simulink model "DDPG"  (R2023a)
settings: Solver=VariableStepAuto  StartTime=0.0  StopTime=10  FixedStep=0.002  RelTol=1e-3
values from neighbouring files (symbols this model uses):
  A = [0 1 0 -1 ... (first row only)    [DDPG_TRAIN.m]
  B = [0; 1/ms; 0; -1/mus]    [DDPG_TRAIN.m]
  B1 = [0; 0; -1; cus/mus]    [DDPG_TRAIN.m]
  C = [1 0 0 0 ... (first row only)    [DDPG_TRAIN.m]
  D = [0; 1/ms]    [DDPG_TRAIN.m]
  Ts = 0.2    [DDPG_TRAIN.m]
undefined symbols (not defined in the file or in its folder): DiscIntNeverNeededParam
libraries: simulink x4, rllib x1
settings Model: Creator=msalm  LastModifiedBy=msalm
settings DataIOCC: ReturnWorkspaceOutputs=off
settings DebuggingCC: AlgebraicLoopMsg=none

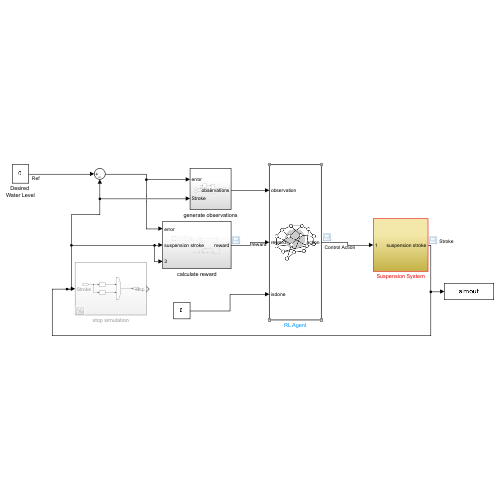
[thumbnail: Simulink's stored preview of the top-level diagram]
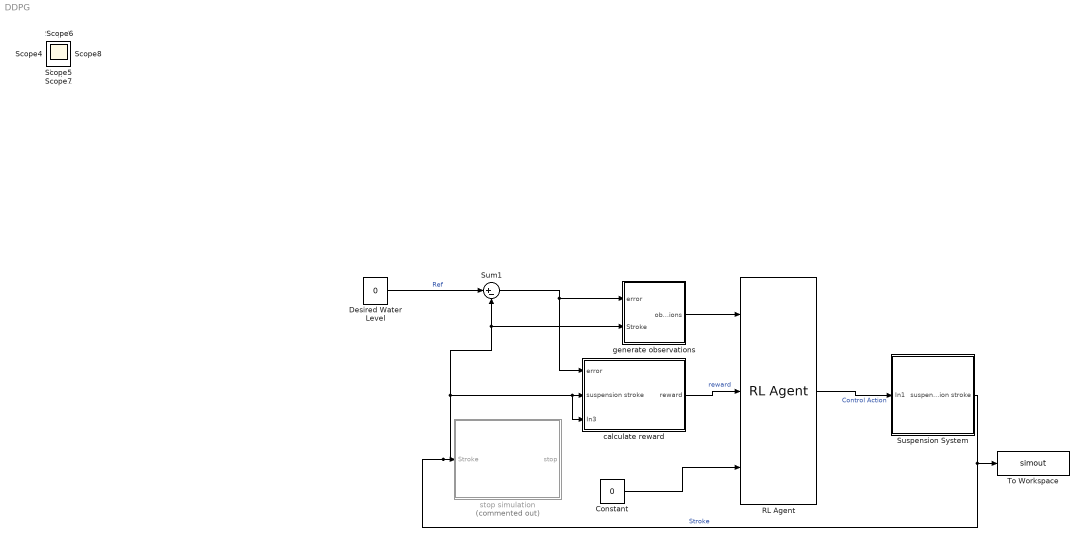
== system DDPG ==
  Constant : Constant  Value=0
  Desired Water Level : Constant  Value=0
  RL Agent : rllib/RL Agent  Agent=agent  ExternalActionAsInput=off  ProvideLastAction=off  ProvideCumRwd=off  TreatAsDirectFeedthrough=on  UseStrictObservationDataTypes=off
  Sum1 : Sum  Inputs=|+-  SaturateOnIntegerOverflow=on
  Suspension System : Subsystem
  To Workspace : ToWorkspace  VariableName=simout  SaveFormat=Timeseries  SampleTime=-1
  calculate reward : Subsystem
  generate observations : Subsystem
  stop simulation : Subsystem  Commented=on
  Scope{,1..8} (9 alike) : Scope
  wires:
  generate observations/1(observations) -> RL Agent/1
  calculate reward/1(reward) -> RL Agent/2  "reward"
  RL Agent/1 -> Suspension System/1(In1)  "Control Action"
  Sum1/1 -> calculate reward/1(error), generate observations/1(error)
  Suspension System/1(suspension stroke) -> stop simulation/1(Stroke), Sum1/2, generate observations/2(Stroke), calculate reward/3(In3), calculate reward/2(suspension stroke), To Workspace/1  "Stroke"
  Desired Water Level/1 -> Sum1/1  "Ref"
  Constant/1 -> RL Agent/3

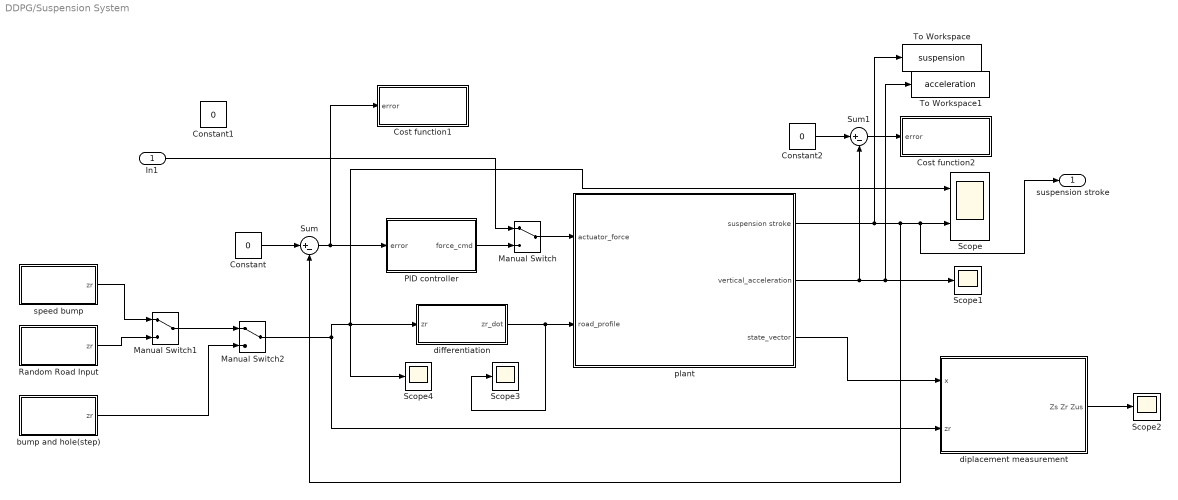
== system DDPG/Suspension System ==
  In1 : Inport
  Constant : Constant  Value=0
  Constant1 : Constant  Value=0
  Constant2 : Constant  Value=0
  Cost function1 : Subsystem
  Cost function2 : Subsystem
  Manual Switch : ManualSwitch
  Manual Switch1 : ManualSwitch
  Manual Switch2 : ManualSwitch
  PID controller : Subsystem
  Random Road Input : Subsystem
  Scope : Scope  NumInputPorts=2
  Scope{1..4} (4 alike) : Scope
  Sum : Sum  Inputs=|+-
  Sum1 : Sum  Inputs=|+-
  To Workspace : ToWorkspace  VariableName=suspension  SampleTime=-1
  To Workspace1 : ToWorkspace  VariableName=acceleration  SampleTime=-1
  bump and hole(step) : Subsystem
  differentiation : Subsystem
  diplacement measurement : Subsystem
  plant : Subsystem
  speed bump : Subsystem
  suspension stroke : Outport
  wires:
  Manual Switch1/1 -> Manual Switch2/1
  plant/3(state_vector) -> diplacement measurement/1(x)
  Random Road Input/1(zr) -> Manual Switch1/2
  Sum1/1 -> Cost function2/1(error)
  Constant2/1 -> Sum1/1
  diplacement measurement/1(Zs Zr Zus) -> Scope2/1
  Constant/1 -> Sum/1
  Sum/1 -> Cost function1/1(error), PID controller/1(error)
  PID controller/1(force_cmd) -> Manual Switch/2
  plant/1(suspension stroke) -> To Workspace/1, Sum/2, suspension stroke/1, Scope/2
  plant/2(vertical_acceleration) -> To Workspace1/1, Scope1/1, Sum1/2
  differentiation/1(zr_dot) -> Scope3/1, plant/2(road_profile)
  Manual Switch/1 -> plant/1(actuator_force)
  bump and hole(step)/1(zr) -> Manual Switch2/2
  speed bump/1(zr) -> Manual Switch1/1
  In1/1 -> Manual Switch/1
  Manual Switch2/1 -> diplacement measurement/2(zr), Scope4/1, Scope/1, differentiation/1(zr)

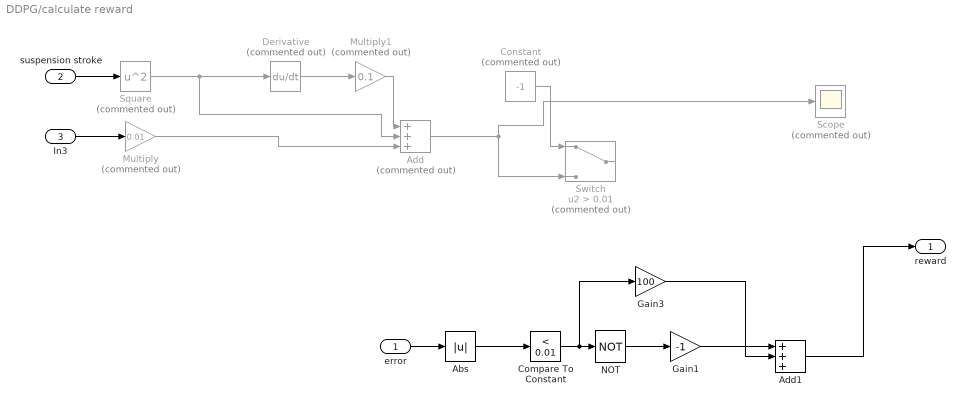
== system DDPG/calculate reward ==
  error : Inport
  suspension stroke : Inport  Port=2
  In3 : Inport  Port=3
  Abs : Abs  SaturateOnIntegerOverflow=off
  Add : Sum  Commented=on  Inputs=+++
  Add1 : Sum  Inputs=+++
  Compare To Constant : simulink/Logic and Bit Operations/Compare To Constant  relop=<  const=0.01  OutDataTypeStr=boolean
  Constant : Constant  Commented=on  Value=-1
  Derivative : Derivative  Commented=on
  Gain1 : Gain  Gain=-1
  Gain3 : Gain  Gain=100
  Multiply : Gain  Commented=on  Gain=0.01
  Multiply1 : Gain  Commented=on  Gain=0.1
  NOT : Logic  Operator=NOT  IconShape=distinctive  AllPortsSameDT=off  OutDataTypeStr=boolean
  Scope : Scope  Commented=on
  Square : Math  Commented=on  Operator=square
  Switch : Switch  Commented=on  Criteria=u2 > Threshold  Threshold=0.01  SaturateOnIntegerOverflow=off  InputSameDT=off
  reward : Outport  VectorParamsAs1DForOutWhenUnconnected=off
  wires:
  Abs/1 -> Compare To Constant/1
  Compare To Constant/1 -> Gain3/1, NOT/1
  Gain1/1 -> Add1/1
  NOT/1 -> Gain1/1
  error/1 -> Abs/1
  suspension stroke/1 -> Square/1
  Square/1 -> Add/2, Derivative/1
  Derivative/1 -> Multiply1/1
  In3/1 -> Multiply/1
  Multiply/1 -> Add/3
  Multiply1/1 -> Add/1
  Add/1 -> Switch/3, Scope/1
  Constant/1 -> Switch/1
  Gain3/1 -> Add1/2
  Add1/1 -> reward/1

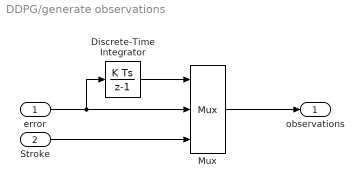
== system DDPG/generate observations ==
  error : Inport
  Stroke : Inport  Port=2
  Discrete-Time Integrator : DiscreteIntegrator  SampleTime=Ts  ICPrevOutput=DiscIntNeverNeededParam  ICPrevScaledInput=DiscIntNeverNeededParam
  Mux : Mux  Inputs=3
  observations : Outport  VectorParamsAs1DForOutWhenUnconnected=off
  wires:
  Stroke/1 -> Mux/3
  Discrete-Time Integrator/1 -> Mux/1
  error/1 -> Discrete-Time Integrator/1, Mux/2
  Mux/1 -> observations/1

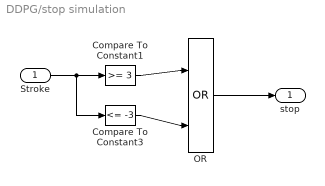
== system DDPG/stop simulation ==
  Stroke : Inport
  Compare To Constant1 : simulink/Logic and Bit Operations/Compare To Constant  relop=>=  const=3  OutDataTypeStr=boolean
  Compare To Constant3 : simulink/Logic and Bit Operations/Compare To Constant  relop=<=  const=-3  OutDataTypeStr=boolean
  OR : Logic  Operator=OR  IconShape=distinctive  AllPortsSameDT=off  OutDataTypeStr=boolean
  stop : Outport  VectorParamsAs1DForOutWhenUnconnected=off
  wires:
  Stroke/1 -> Compare To Constant3/1, Compare To Constant1/1
  Compare To Constant3/1 -> OR/2
  Compare To Constant1/1 -> OR/1
  OR/1 -> stop/1

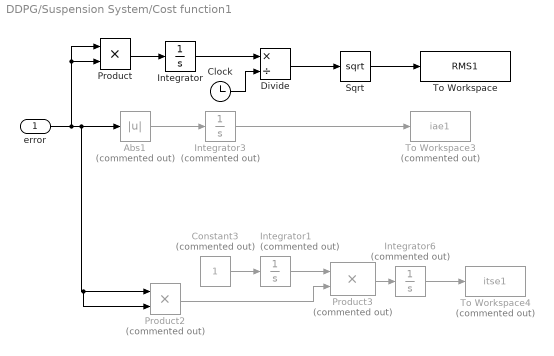
== system DDPG/Suspension System/Cost function1 ==
  error : Inport
  Abs1 : Abs  Commented=on
  Clock : Clock
  Constant3 : Constant  Commented=on
  Divide : Product  Inputs=*/
  Integrator : Integrator
  Integrator1 : Integrator  Commented=on
  Integrator3 : Integrator  Commented=on
  Integrator6 : Integrator  Commented=on
  Product : Product
  Product2 : Product  Commented=on
  Product3 : Product  Commented=on  SaturateOnIntegerOverflow=on  OutDataTypeStr=Inherit: Same as first input
  Sqrt : Sqrt
  To Workspace : ToWorkspace  VariableName=RMS1  SampleTime=-1
      settings: MaxDataPoints=1
  To Workspace3 : ToWorkspace  Commented=on  VariableName=iae1  SampleTime=-1
      settings: MaxDataPoints=1
  To Workspace4 : ToWorkspace  Commented=on  VariableName=itse1  SampleTime=-1
      settings: MaxDataPoints=1
  wires:
  Integrator3/1 -> To Workspace3/1
  error/1 -> Product/2, Product/1, Product2/2, Product2/1, Abs1/1
  Abs1/1 -> Integrator3/1
  Integrator1/1 -> Product3/1
  Constant3/1 -> Integrator1/1
  Product2/1 -> Product3/2
  Integrator6/1 -> To Workspace4/1
  Product3/1 -> Integrator6/1
  Product/1 -> Integrator/1
  Integrator/1 -> Divide/1
  Clock/1 -> Divide/2
  Divide/1 -> Sqrt/1
  Sqrt/1 -> To Workspace/1

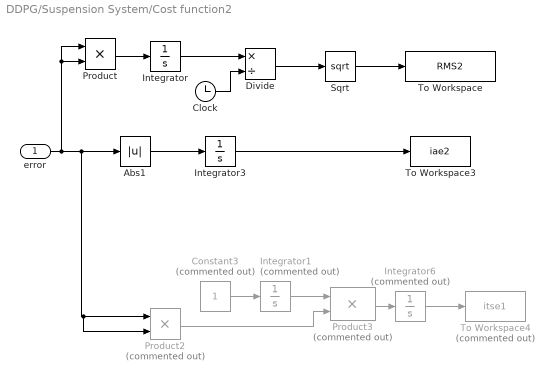
== system DDPG/Suspension System/Cost function2 ==
  error : Inport
  Abs1 : Abs
  Clock : Clock
  Constant3 : Constant  Commented=on
  Divide : Product  Inputs=*/
  Integrator : Integrator
  Integrator1 : Integrator  Commented=on
  Integrator3 : Integrator
  Integrator6 : Integrator  Commented=on
  Product : Product
  Product2 : Product  Commented=on
  Product3 : Product  Commented=on  SaturateOnIntegerOverflow=on  OutDataTypeStr=Inherit: Same as first input
  Sqrt : Sqrt
  To Workspace : ToWorkspace  VariableName=RMS2  SampleTime=-1
      settings: MaxDataPoints=1
  To Workspace3 : ToWorkspace  VariableName=iae2  SampleTime=-1
      settings: MaxDataPoints=1
  To Workspace4 : ToWorkspace  Commented=on  VariableName=itse1  SampleTime=-1
      settings: MaxDataPoints=1
  wires:
  Integrator3/1 -> To Workspace3/1
  error/1 -> Product/2, Product/1, Product2/2, Product2/1, Abs1/1
  Abs1/1 -> Integrator3/1
  Integrator1/1 -> Product3/1
  Constant3/1 -> Integrator1/1
  Product2/1 -> Product3/2
  Integrator6/1 -> To Workspace4/1
  Product3/1 -> Integrator6/1
  Clock/1 -> Divide/2
  Sqrt/1 -> To Workspace/1
  Product/1 -> Integrator/1
  Divide/1 -> Sqrt/1
  Integrator/1 -> Divide/1

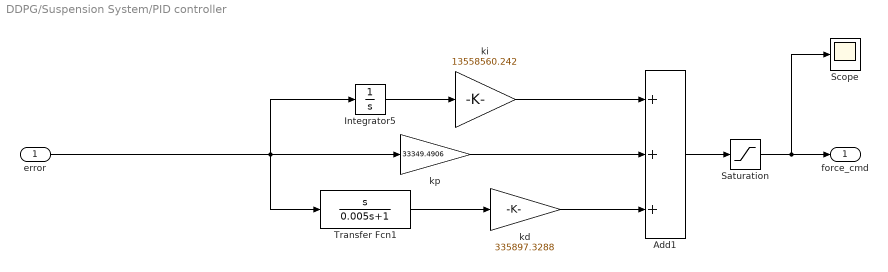
== system DDPG/Suspension System/PID controller ==
  error : Inport
  Add1 : Sum  Inputs=+++
  Integrator5 : Integrator
  Saturation : Saturate  UpperLimit=2000  LowerLimit=-2000
  Scope : Scope
  Transfer Fcn1 : TransferFcn  Numerator=[1 0]  Denominator=[0.005 1]
  kd : Gain  Gain=335897.3288
  ki : Gain  Gain=13558560.242
  kp : Gain  Gain=33349.4906
  force_cmd : Outport
  wires:
  kd/1 -> Add1/3
  kp/1 -> Add1/2
  Transfer Fcn1/1 -> kd/1
  Integrator5/1 -> ki/1
  error/1 -> Transfer Fcn1/1, kp/1, Integrator5/1
  ki/1 -> Add1/1
  Add1/1 -> Saturation/1
  Saturation/1 -> Scope/1, force_cmd/1

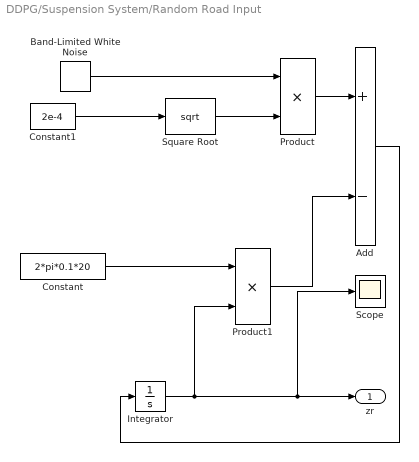
== system DDPG/Suspension System/Random Road Input ==
  Add : Sum  Inputs=+-
  Band-Limited White Noise : simulink/Sources/Band-Limited White Noise  Cov=[0.1]  Ts=0.002  seed=[23341]
  Constant : Constant  Value=2*pi*0.1*20
  Constant1 : Constant  Value=2e-4
  Integrator : Integrator
  Product : Product
  Product1 : Product
  Scope : Scope
  Square Root : Sqrt
  zr : Outport
  wires:
  Band-Limited White Noise/1 -> Product/1
  Product/1 -> Add/1
  Product1/1 -> Add/2
  Integrator/1 -> Scope/1, zr/1, Product1/2
  Add/1 -> Integrator/1
  Constant/1 -> Product1/1
  Square Root/1 -> Product/2
  Constant1/1 -> Square Root/1

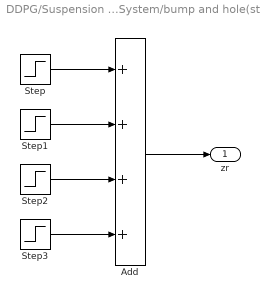
== system DDPG/Suspension System/bump and hole(step) ==
  Add : Sum  Inputs=++++
  Step : Step  After=0.05  SampleTime=0
  Step1 : Step  Time=2  After=-0.05  SampleTime=0
  Step2 : Step  Time=5  After=-0.05  SampleTime=0
  Step3 : Step  Time=6  After=0.05  SampleTime=0
  zr : Outport
  wires:
  Step3/1 -> Add/4
  Step2/1 -> Add/3
  Step/1 -> Add/1
  Step1/1 -> Add/2
  Add/1 -> zr/1

== system DDPG/Suspension System/differentiation ==
  zr : Inport
  Derivative : Derivative
  Transfer Fcn : TransferFcn  Denominator=[0.01 1]
  zr_dot : Outport
  wires:
  zr/1 -> Transfer Fcn/1
  Transfer Fcn/1 -> Derivative/1
  Derivative/1 -> zr_dot/1

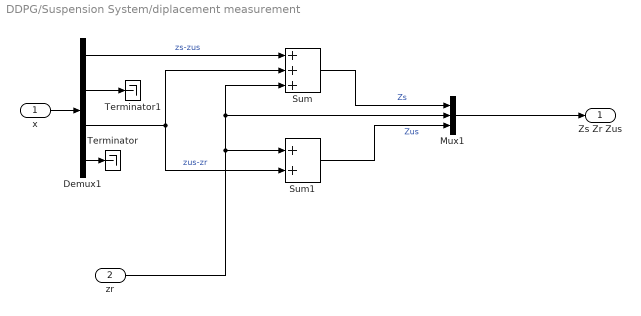
== system DDPG/Suspension System/diplacement measurement ==
  x : Inport
  zr : Inport  Port=2
  Demux1 : Demux
  Mux1 : Mux  Inputs=3
  Sum : Sum  Inputs=+++
  Sum1 : Sum
  Terminator : Terminator
  Terminator1 : Terminator
  Zs Zr Zus : Outport
  wires:
  Demux1/2 -> Terminator1/1
  Demux1/4 -> Terminator/1
  Demux1/1 -> Sum/1  "zs-zus"
  Demux1/3 -> Sum1/2, Sum/2  "zus-zr"
  Sum/1 -> Mux1/1  "Zs"
  Sum1/1 -> Mux1/3  "Zus"
  Mux1/1 -> Zs Zr Zus/1
  zr/1 -> Sum1/1, Mux1/2, Sum/3
  x/1 -> Demux1/1

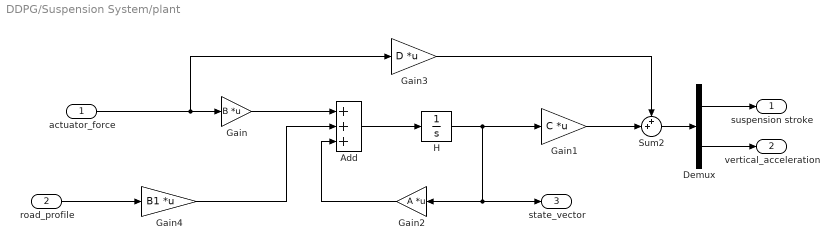
== system DDPG/Suspension System/plant ==
  actuator_force : Inport
  road_profile : Inport  Port=2
  Add : Sum  Inputs=+++
  Demux : Demux  Outputs=2
  Gain : Gain  Gain=B  Multiplication=Matrix(K*u)
  Gain1 : Gain  Gain=C  Multiplication=Matrix(K*u)
  Gain2 : Gain  Gain=A  Multiplication=Matrix(K*u)
  Gain3 : Gain  Gain=D  Multiplication=Matrix(K*u)
  Gain4 : Gain  Gain=B1  Multiplication=Matrix(K*u)
  H : Integrator  UpperSaturationLimit=3  LowerSaturationLimit=0
  Sum2 : Sum  Inputs=++|
  suspension stroke : Outport
  vertical_acceleration : Outport  Port=2
  state_vector : Outport  Port=3
  wires:
  H/1 -> Gain1/1, Gain2/1, state_vector/1
  Gain1/1 -> Sum2/2
  actuator_force/1 -> Gain3/1, Gain/1
  Gain3/1 -> Sum2/1
  road_profile/1 -> Gain4/1
  Add/1 -> H/1
  Gain/1 -> Add/1
  Gain2/1 -> Add/3
  Gain4/1 -> Add/2
  Sum2/1 -> Demux/1
  Demux/1 -> suspension stroke/1
  Demux/2 -> vertical_acceleration/1

== system DDPG/Suspension System/speed bump ==
  Product : Product
  Pulse Generator : DiscretePulseGenerator  PulseType=Time based  Period=3  PulseWidth=10/3  PhaseDelay=2
  Sine Wave : Sin  Amplitude=0.08  Frequency=10*pi
  zr : Outport
  wires:
  Sine Wave/1 -> Product/2
  Pulse Generator/1 -> Product/1
  Product/1 -> zr/1
